simulink model "planLocalPathTEB"  (R2024b)
settings: Solver=FixedStepDiscrete  StartTime=0.0  StopTime=10.0  RelTol=1e-3
undefined symbols (not defined in the file or in its folder): fixedControllerParams, maxLocalPathLen, maxRefPathLen
settings Model: DataDictionary=LocalPlannerTEBData.sldd  Creator=cstabile  LastModifiedBy=apattass
settings SFSimCC: SimTargetLang=C++

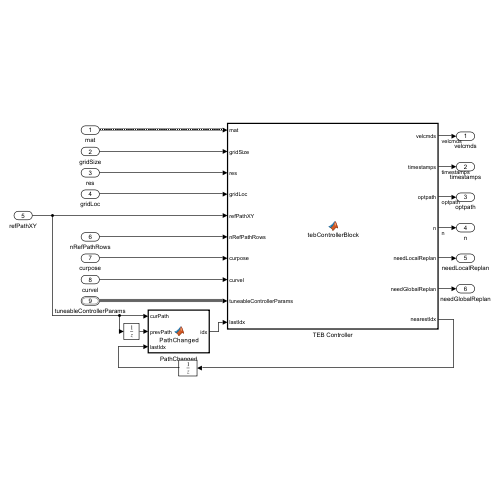
[thumbnail: Simulink's stored preview of the top-level diagram]
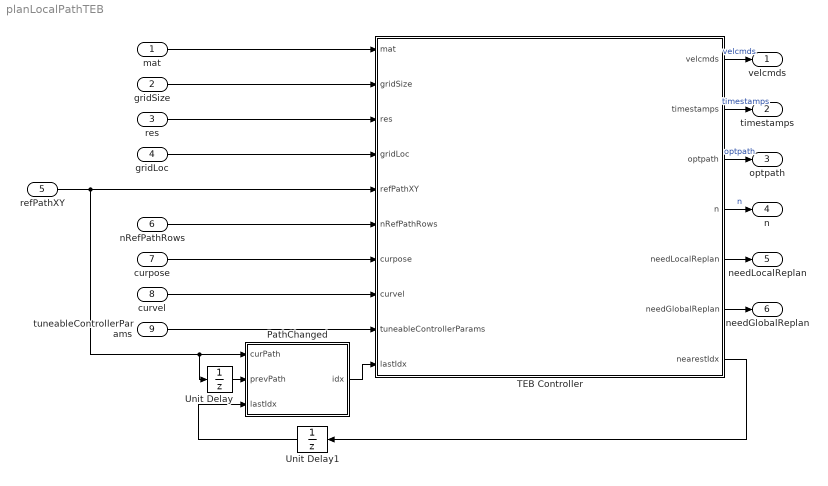
== system planLocalPathTEB ==
  mat : Inport  OutDataTypeStr=boolean  PortDimensions=[1201 1201]  Interpolate=off
      settings: VarSizeSig=Yes
  gridSize : Inport  Port=2
  res : Inport  Port=3
  gridLoc : Inport  Port=4
  refPathXY : Inport  Port=5  PortDimensions=[maxRefPathLen 3]  Interpolate=off
  nRefPathRows : Inport  Port=6
  curpose : Inport  Port=7
  curvel : Inport  Port=8
  tuneableControllerParams : Inport  Port=9  OutDataTypeStr=Bus: controller_bus
  PathChanged : MATLAB Function  TreatAsAtomicUnit=on
  TEB Controller : MATLAB Function  TreatAsAtomicUnit=on  mask{length=fixedControllerParams.Length, width=fixedControllerParams.Width, numIteration=fixedControllerParams.NumIteration, referenceDeltaTime=fixedControllerParams.ReferenceDeltaTime, nRowOutput=maxLocalPathLen}
      mask prompts: length "Length of vehicle (in meters)"; width "Width of vehicle (in meters)"; numIteration "Number of optimization iterations per call"; referenceDeltaTime "Desired timespan between control commands (in seconds)"; nRowOutput "MaxNumOutput"
  Unit Delay : UnitDelay  SampleTime=-1  HasFrameUpgradeWarning=on
  Unit Delay1 : UnitDelay  SampleTime=-1  HasFrameUpgradeWarning=on
  velcmds : Outport  OutDataTypeStr=double  PortDimensions=[1000 2]
  timestamps : Outport  Port=2  OutDataTypeStr=double  PortDimensions=[1000 1]
  optpath : Outport  Port=3  OutDataTypeStr=double  PortDimensions=[1000 3]
  n : Outport  Port=4  OutDataTypeStr=double  PortDimensions=1
  needLocalReplan : Outport  Port=5  OutDataTypeStr=boolean  PortDimensions=1
  needGlobalReplan : Outport  Port=6  OutDataTypeStr=boolean  PortDimensions=1
  wires:
  gridSize/1 -> TEB Controller/2(gridSize)
  curpose/1 -> TEB Controller/7(curpose)
  tuneableControllerParams/1 -> TEB Controller/9(tuneableControllerParams)
  curvel/1 -> TEB Controller/8(curvel)
  refPathXY/1 -> TEB Controller/5(refPathXY), PathChanged/1(curPath), Unit Delay/1
  mat/1 -> TEB Controller/1(mat)
  nRefPathRows/1 -> TEB Controller/6(nRefPathRows)
  gridLoc/1 -> TEB Controller/4(gridLoc)
  TEB Controller/3(optpath) -> optpath/1  "optpath"
  TEB Controller/6(needGlobalReplan) -> needGlobalReplan/1
  TEB Controller/4(n) -> n/1  "n"
  TEB Controller/5(needLocalReplan) -> needLocalReplan/1
  TEB Controller/1(velcmds) -> velcmds/1  "velcmds"
  TEB Controller/2(timestamps) -> timestamps/1  "timestamps"
  res/1 -> TEB Controller/3(res)
  Unit Delay/1 -> PathChanged/2(prevPath)
  PathChanged/1(idx) -> TEB Controller/10(lastIdx)
  TEB Controller/7(nearestIdx) -> Unit Delay1/1
  Unit Delay1/1 -> PathChanged/3(lastIdx)

== matlab function planLocalPathTEB/PathChanged ==
  data: curPath input; prevPath input; lastIdx input; idx output
function idx = PathChanged(curPath, prevPath, lastIdx)
%PathChanged Reset the nearest index when new path has been provided
    if ~isequal(curPath,prevPath)
        idx = 1;
    else
        idx = lastIdx;
    end
end

== matlab function planLocalPathTEB/TEB Controller ==
  data: mat input; gridSize input size=[1 2]; res input; velcmds output size=[nRowOutput 2]; gridLoc input size=[1 2]; refPathXY input size=[maxRefPathLen 3]; nRefPathRows input; curpose input size=[1 3]; curvel input size=[1 2]; tuneableControllerParams input Bus: controller_bus; timestamps output size=[nRowOutput 1]; optpath output size=[nRowOutput 3]; length parameter; width parameter; numIteration parameter; referenceDeltaTime parameter; n output size=[1 1]; nRowOutput parameter; needLocalReplan output; needGlobalReplan output; lastIdx input; nearestIdx output
function [velcmds,timestamps,optpath,n,needLocalReplan,needGlobalReplan,nearestIdx] = tebControllerBlock(mat, gridSize, res, ...
    gridLoc, refPathXY, nRefPathRows, curpose, curvel, tuneableControllerParams, ...
    length, width, numIteration, referenceDeltaTime, nRowOutput, lastIdx)
    
    velcmds = nan(nRowOutput,2);
    timestamps = nan(nRowOutput,1);
    optpath = nan(nRowOutput,3);
    n = 0;
    needLocalReplan = false;
    needGlobalReplan = false;
    nearestIdx = 1;
    if nRefPathRows ~= 0
        egoMat = mat(1:gridSize(1),1:gridSize(2));

        [velcmds_,timestamps_,optpath_,nearestIdx,~,needLocalReplan,needGlobalReplan] = TEBControllerFcn(egoMat, res, gridLoc, ...
            refPathXY(1:nRefPathRows,:), lastIdx, curpose, curvel, tuneableControllerParams, ...
            length, width, numIteration, referenceDeltaTime);

        n = numel(timestamps_);
        velcmds(1:n,:)      = velcmds_;
        timestamps(1:n,:)   = timestamps_;
        optpath(1:n,:)      = optpath_;
    end
end
